simulink library "halin"  (R2021b)
settings: Solver=VariableStepAuto  StartTime=0.0  StopTime=10.0  RelTol=1e-3
undefined symbols (not defined in the file): KHAL_CAN1ABM1E2E_flg, KHAL_CAN1EPB1E2E_flg, KHAL_CAN1EPS1E2E_flg, KHAL_CAN1ESC1E2E_flg, KHAL_CAN1ESC5E2E_flg, KHAL_CAN3BMS1E2E_flg, KHAL_CAN3BMS6E2E_flg, KHAL_CAN3CCU1E2E_flg, KHAL_CAN3CCU2E2E_flg, KHAL_CAN3MCUNF1E2E_flg, KHAL_CAN3MCUNR1E2E_flg, KHAL_CAN3Shifter1E2E_flg, KHAL_CAN3Shifter2E2E_flg, KHAL_CAN6FCM2E2E_flg, KHAL_CAN6FCM4E2E_flg, TRUE
libraries: simulink x645, FVT_lib x207, hcu_lib x59
(part 6 of 23)

== system halin/HAL_IN/CAN1/EPS1 ==
  DT_CAN1_SG_EPS1 : Inport
  0x8E : Constant  Value=0x8E
  0xB1 : Constant  Value=0xB1
  BitwiseAND{,1..34} (35 alike) : simulink/Logic and Bit Operations/Bitwise Operator  logicop=AND  UseBitMask=on  BitMask=0xFF  BitMaskRealWorld=Stored Integer
  BitwiseOR{,1,4..6,8..10,12,14..15} (11 alike) : simulink/Logic and Bit Operations/Bitwise Operator  logicop=OR  UseBitMask=off  BitMask=bin2dec('11011001')  BitMaskRealWorld=Stored Integer
  BitwiseOR11 : simulink/Logic and Bit Operations/Bitwise Operator  logicop=OR  UseBitMask=off  NumInputPorts=6  BitMask=bin2dec('11011001')  BitMaskRealWorld=Stored Integer
  BitwiseOR13 : simulink/Logic and Bit Operations/Bitwise Operator  logicop=OR  UseBitMask=off  NumInputPorts=3  BitMask=bin2dec('11011001')  BitMaskRealWorld=Stored Integer
  BitwiseOR2 : simulink/Logic and Bit Operations/Bitwise Operator  logicop=OR  UseBitMask=off  NumInputPorts=6  BitMask=bin2dec('11011001')  BitMaskRealWorld=Stored Integer
  BitwiseOR3 : simulink/Logic and Bit Operations/Bitwise Operator  logicop=OR  UseBitMask=off  NumInputPorts=3  BitMask=bin2dec('11011001')  BitMaskRealWorld=Stored Integer
  BitwiseOR7 : simulink/Logic and Bit Operations/Bitwise Operator  logicop=OR  UseBitMask=off  NumInputPorts=6  BitMask=bin2dec('11011001')  BitMaskRealWorld=Stored Integer
  DDM_CS&RC_Comparison : FVT_lib/hal/DDM_CS&RC_Comparison  MsgCycleTime=10
  Data Type Conversion{,1..34} (35 alike) : DataTypeConversion  OutDataTypeStr=uint8
  DriIntend : Subsystem
  EPSAOIControl : Subsystem
  EPSRC : Subsystem
  EPSTOIActivation : Subsystem
  EPSTOIFault : Subsystem
  EPSTOIUnavailable : Subsystem
  EpasFailed : Subsystem
  KHAL_CAN1EPS1E2E_flg : Constant  Value=KHAL_CAN1EPS1E2E_flg
  LeftShift{,2,6..7} (4 alike) : ArithShift  BitShiftNumber=1  BitShiftDirection=Left
  LeftShift1 : ArithShift  BitShiftNumber=3  BitShiftDirection=Left
  LeftShift10 : ArithShift  BitShiftNumber=3  BitShiftDirection=Left
  LeftShift{3..4,11,15,17,21,23} (7 alike) : ArithShift  BitShiftDirection=Left
  LeftShift12 : ArithShift  BitShiftNumber=5  BitShiftDirection=Left
  LeftShift13 : ArithShift  BitShiftNumber=7  BitShiftDirection=Left
  LeftShift14 : ArithShift  BitShiftNumber=6  BitShiftDirection=Left
  LeftShift16 : ArithShift  BitShiftNumber=5  BitShiftDirection=Left
  LeftShift18 : ArithShift  BitShiftNumber=4  BitShiftDirection=Left
  LeftShift19 : ArithShift  BitShiftNumber=6  BitShiftDirection=Left
  LeftShift20 : ArithShift  BitShiftNumber=7  BitShiftDirection=Left
  LeftShift22 : ArithShift  BitShiftNumber=6  BitShiftDirection=Left
  LeftShift24 : ArithShift  BitShiftNumber=4  BitShiftDirection=Left
  LeftShift5 : ArithShift  BitShiftNumber=2  BitShiftDirection=Left
  LeftShift8 : ArithShift  BitShiftNumber=3  BitShiftDirection=Left
  LeftShift9 : ArithShift  BitShiftNumber=5  BitShiftDirection=Left
  MessageRollingCounter : FVT_lib/hal/MessageRollingCounter  CounterMAX=14  task_time_ms=5  msg_time_ms=10
  Mux : Mux  Inputs=15
  RightShift{,2,6,8} (4 alike) : ArithShift  BitShiftNumber=8
  RightShift{1,3,7,9} (4 alike) : ArithShift
  RightShift4 : ArithShift  BitShiftNumber=3
  RightShift5 : ArithShift  BitShiftNumber=-5
  SASAngle : Subsystem
  SASCAL : Subsystem
  SASSpeed : Subsystem
  SASSpeedValid : Subsystem
  SASV : Subsystem
  bus_selector : BusSelector  OutputSignals=CAN1_DriIntend,CAN1_EPS_AOI_Control,CAN1_EPS_AOI_Dis_R,CAN1_EPS_CS,CAN1_EPS_DMSMode_Sta,CAN1_EPS_ESABoostOut_Trq,CAN1_EPS_ESAInpBoost_Sta,CAN1_EPS_LDW_Activation,CAN1_EPS_LDW_Unavailable,CAN1_EPS_Pwr_Consumpt,CAN1_EPS_Pwr_Consumpt_V,CAN1_EPS_Pwr_Limit,CAN1_EPS_Pwr_Limit_V,CAN1_EPS_RC,CAN1_EPS_TOI_Activation,CAN1_EPS_TOI_Dis_R,CAN1_EPS_TOI_Fault,CAN1_EPS_TOI_Unavailable,CAN1_EPS_Temp,CAN1_EPS_Temp_V,CAN1_EPS_VOL,CAN1_EPS_VOL_V,CAN1_EpasFailed,CAN1_SAS_Angle,CAN1_SAS_CAL,CAN1_SAS_Speed,CAN1_SAS_Speed_Valid,CAN1_SAS_V,CAN1_Steering_Torque,CAN1_Steering_Torque_V
  bus_selector1 : BusSelector  OutputSignals=CAN1_DriIntend
  bus_selector10 : BusSelector  OutputSignals=CAN1_SAS_Speed
  bus_selector11 : BusSelector  OutputSignals=CAN1_SAS_Speed_Valid
  bus_selector12 : BusSelector  OutputSignals=CAN1_SAS_V
  bus_selector2 : BusSelector  OutputSignals=CAN1_EPS_AOI_Control
  bus_selector3 : BusSelector  OutputSignals=CAN1_EPS_RC
  bus_selector4 : BusSelector  OutputSignals=CAN1_EPS_TOI_Activation
  bus_selector5 : BusSelector  OutputSignals=CAN1_EPS_TOI_Fault
  bus_selector6 : BusSelector  OutputSignals=CAN1_EPS_TOI_Unavailable
  bus_selector7 : BusSelector  OutputSignals=CAN1_EpasFailed
  bus_selector8 : BusSelector  OutputSignals=CAN1_SAS_Angle
  bus_selector9 : BusSelector  OutputSignals=CAN1_SAS_CAL
  VHAL_EPS1CSErr_flg : Outport
  VHAL_EPS1RCErr_flg : Outport  Port=2
  VHAL_DriIntend_enum : Outport  Port=3
  VHAL_EPSAOIControl_enum : Outport  Port=4
  VHAL_EPSRC_enum : Outport  Port=5
  VHAL_EPSTOIActivation_flg : Outport  Port=6
  VHAL_EPSTOIFault_flg : Outport  Port=7
  VHAL_EPSTOIUnavailable_flg : Outport  Port=8
  VHAL_EpasFailed_enum : Outport  Port=9
  VHAL_SASAngle_Deg : Outport  Port=10
  VHAL_SASCAL_flg : Outport  Port=11
  VHAL_SASSpeed_degps : Outport  Port=12
  VHAL_SASSpeedValid_flg : Outport  Port=13
  VHAL_SASV_flg : Outport  Port=14
  wires:
  DT_CAN1_SG_EPS1/1 -> [DT_CAN1_SG_EPS1]
  [DT_CAN1_SG_EPS1] -> bus_selector/1
  bus_selector/1 -> [CAN1_DriIntend]  "<CAN1_DriIntend>"
  [CAN1_DriIntend] -> LeftShift/1
  LeftShift/1 -> BitwiseAND/1
  BitwiseAND/1 -> [Byte_2_CAN1_DriIntend]
  bus_selector/2 -> [CAN1_EPS_AOI_Control]  "<CAN1_EPS_AOI_Control>"
  [CAN1_EPS_AOI_Control] -> LeftShift1/1
  LeftShift1/1 -> BitwiseAND1/1
  BitwiseAND1/1 -> [Byte_2_CAN1_EPS_AOI_Control]
  bus_selector/3 -> [CAN1_EPS_AOI_Dis_R]  "<CAN1_EPS_AOI_Dis_R>"
  [CAN1_EPS_AOI_Dis_R] -> LeftShift2/1
  LeftShift2/1 -> BitwiseAND2/1
  BitwiseAND2/1 -> [Byte_3_CAN1_EPS_AOI_Dis_R]
  bus_selector/4 -> [CAN1_EPS_CS]  "<CAN1_EPS_CS>"
  [CAN1_EPS_CS] -> LeftShift3/1
  LeftShift3/1 -> BitwiseAND3/1
  BitwiseAND3/1 -> [Byte_0_CAN1_EPS_CS]
  bus_selector/5 -> [CAN1_EPS_DMSMode_Sta]  "<CAN1_EPS_DMSMode_Sta>"
  [CAN1_EPS_DMSMode_Sta] -> LeftShift4/1
  LeftShift4/1 -> BitwiseAND4/1
  BitwiseAND4/1 -> [Byte_15_CAN1_EPS_DMSMode_Sta]
  bus_selector/6 -> [CAN1_EPS_ESABoostOut_Trq]  "<CAN1_EPS_ESABoostOut_Trq>"
  [CAN1_EPS_ESABoostOut_Trq] -> LeftShift5/1
  LeftShift5/1 -> BitwiseAND5/1
  BitwiseAND5/1 -> [Byte_13_CAN1_EPS_ESABoostOut_Trq]
  bus_selector/7 -> [CAN1_EPS_ESAInpBoost_Sta]  "<CAN1_EPS_ESAInpBoost_Sta>"
  [CAN1_EPS_ESAInpBoost_Sta] -> LeftShift6/1
  LeftShift6/1 -> BitwiseAND6/1
  BitwiseAND6/1 -> [Byte_13_CAN1_EPS_ESAInpBoost_Sta]
  bus_selector/8 -> [CAN1_EPS_LDW_Activation]  "<CAN1_EPS_LDW_Activation>"
  [CAN1_EPS_LDW_Activation] -> LeftShift7/1
  LeftShift7/1 -> BitwiseAND7/1
  BitwiseAND7/1 -> [Byte_11_CAN1_EPS_LDW_Activation]
  bus_selector/9 -> [CAN1_EPS_LDW_Unavailable]  "<CAN1_EPS_LDW_Unavailable>"
  [CAN1_EPS_LDW_Unavailable] -> LeftShift8/1
  LeftShift8/1 -> BitwiseAND8/1
  BitwiseAND8/1 -> [Byte_11_CAN1_EPS_LDW_Unavailable]
  bus_selector/10 -> [CAN1_EPS_Pwr_Consumpt]  "<CAN1_EPS_Pwr_Consumpt>"
  [CAN1_EPS_Pwr_Consumpt] -> RightShift/1, RightShift1/1
  RightShift/1 -> BitwiseAND9/1
  BitwiseAND9/1 -> [Byte_13_CAN1_EPS_Pwr_Consumpt]
  RightShift1/1 -> BitwiseAND10/1
  BitwiseAND10/1 -> [Byte_14_CAN1_EPS_Pwr_Consumpt]
  bus_selector/11 -> [CAN1_EPS_Pwr_Consumpt_V]  "<CAN1_EPS_Pwr_Consumpt_V>"
  [CAN1_EPS_Pwr_Consumpt_V] -> LeftShift9/1
  LeftShift9/1 -> BitwiseAND11/1
  BitwiseAND11/1 -> [Byte_7_CAN1_EPS_Pwr_Consumpt_V]
  bus_selector/12 -> [CAN1_EPS_Pwr_Limit]  "<CAN1_EPS_Pwr_Limit>"
  [CAN1_EPS_Pwr_Limit] -> RightShift2/1, RightShift3/1
  RightShift2/1 -> BitwiseAND12/1
  BitwiseAND12/1 -> [Byte_11_CAN1_EPS_Pwr_Limit]
  RightShift3/1 -> BitwiseAND13/1
  BitwiseAND13/1 -> [Byte_12_CAN1_EPS_Pwr_Limit]
  bus_selector/13 -> [CAN1_EPS_Pwr_Limit_V]  "<CAN1_EPS_Pwr_Limit_V>"
  [CAN1_EPS_Pwr_Limit_V] -> LeftShift10/1
  LeftShift10/1 -> BitwiseAND14/1
  BitwiseAND14/1 -> [Byte_7_CAN1_EPS_Pwr_Limit_V]
  bus_selector/14 -> [CAN1_EPS_RC]  "<CAN1_EPS_RC>"
  [CAN1_EPS_RC] -> LeftShift11/1
  LeftShift11/1 -> BitwiseAND15/1
  BitwiseAND15/1 -> [Byte_1_CAN1_EPS_RC]
  bus_selector/15 -> [CAN1_EPS_TOI_Activation]  "<CAN1_EPS_TOI_Activation>"
  [CAN1_EPS_TOI_Activation] -> LeftShift12/1
  LeftShift12/1 -> BitwiseAND16/1
  BitwiseAND16/1 -> [Byte_2_CAN1_EPS_TOI_Activation]
  bus_selector/16 -> [CAN1_EPS_TOI_Dis_R]  "<CAN1_EPS_TOI_Dis_R>"
  [CAN1_EPS_TOI_Dis_R] -> RightShift4/1, RightShift5/1
  RightShift4/1 -> BitwiseAND17/1
  BitwiseAND17/1 -> [Byte_2_CAN1_EPS_TOI_Dis_R]
  RightShift5/1 -> BitwiseAND18/1
  BitwiseAND18/1 -> [Byte_3_CAN1_EPS_TOI_Dis_R]
  bus_selector/17 -> [CAN1_EPS_TOI_Fault]  "<CAN1_EPS_TOI_Fault>"
  [CAN1_EPS_TOI_Fault] -> LeftShift13/1
  LeftShift13/1 -> BitwiseAND19/1
  BitwiseAND19/1 -> [Byte_2_CAN1_EPS_TOI_Fault]
  bus_selector/18 -> [CAN1_EPS_TOI_Unavailable]  "<CAN1_EPS_TOI_Unavailable>"
  [CAN1_EPS_TOI_Unavailable] -> LeftShift14/1
  LeftShift14/1 -> BitwiseAND20/1
  BitwiseAND20/1 -> [Byte_2_CAN1_EPS_TOI_Unavailable]
  bus_selector/19 -> [CAN1_EPS_Temp]  "<CAN1_EPS_Temp>"
  [CAN1_EPS_Temp] -> LeftShift15/1
  LeftShift15/1 -> BitwiseAND21/1
  BitwiseAND21/1 -> [Byte_10_CAN1_EPS_Temp]
  bus_selector/20 -> [CAN1_EPS_Temp_V]  "<CAN1_EPS_Temp_V>"
  [CAN1_EPS_Temp_V] -> LeftShift16/1
  LeftShift16/1 -> BitwiseAND22/1
  BitwiseAND22/1 -> [Byte_11_CAN1_EPS_Temp_V]
  bus_selector/21 -> [CAN1_EPS_VOL]  "<CAN1_EPS_VOL>"
  [CAN1_EPS_VOL] -> LeftShift17/1
  LeftShift17/1 -> BitwiseAND23/1
  BitwiseAND23/1 -> [Byte_9_CAN1_EPS_VOL]
  bus_selector/22 -> [CAN1_EPS_VOL_V]  "<CAN1_EPS_VOL_V>"
  [CAN1_EPS_VOL_V] -> LeftShift18/1
  LeftShift18/1 -> BitwiseAND24/1
  BitwiseAND24/1 -> [Byte_11_CAN1_EPS_VOL_V]
  bus_selector/23 -> [CAN1_EpasFailed]  "<CAN1_EpasFailed>"
  [CAN1_EpasFailed] -> LeftShift19/1
  LeftShift19/1 -> BitwiseAND25/1
  BitwiseAND25/1 -> [Byte_11_CAN1_EpasFailed]
  bus_selector/24 -> [CAN1_SAS_Angle]  "<CAN1_SAS_Angle>"
  [CAN1_SAS_Angle] -> RightShift6/1, RightShift7/1
  RightShift6/1 -> BitwiseAND26/1
  BitwiseAND26/1 -> [Byte_5_CAN1_SAS_Angle]
  RightShift7/1 -> BitwiseAND27/1
  BitwiseAND27/1 -> [Byte_6_CAN1_SAS_Angle]
  bus_selector/25 -> [CAN1_SAS_CAL]  "<CAN1_SAS_CAL>"
  [CAN1_SAS_CAL] -> LeftShift20/1
  LeftShift20/1 -> BitwiseAND28/1
  BitwiseAND28/1 -> [Byte_7_CAN1_SAS_CAL]
  bus_selector/26 -> [CAN1_SAS_Speed]  "<CAN1_SAS_Speed>"
  [CAN1_SAS_Speed] -> LeftShift21/1
  LeftShift21/1 -> BitwiseAND29/1
  BitwiseAND29/1 -> [Byte_4_CAN1_SAS_Speed]
  bus_selector/27 -> [CAN1_SAS_Speed_Valid]  "<CAN1_SAS_Speed_Valid>"
  [CAN1_SAS_Speed_Valid] -> LeftShift22/1
  LeftShift22/1 -> BitwiseAND30/1
  BitwiseAND30/1 -> [Byte_7_CAN1_SAS_Speed_Valid]
  bus_selector/28 -> [CAN1_SAS_V]  "<CAN1_SAS_V>"
  [CAN1_SAS_V] -> LeftShift23/1
  LeftShift23/1 -> BitwiseAND31/1
  BitwiseAND31/1 -> [Byte_3_CAN1_SAS_V]
  bus_selector/29 -> [CAN1_Steering_Torque]  "<CAN1_Steering_Torque>"
  [CAN1_Steering_Torque] -> RightShift8/1, RightShift9/1
  RightShift8/1 -> BitwiseAND32/1
  BitwiseAND32/1 -> [Byte_7_CAN1_Steering_Torque]
  RightShift9/1 -> BitwiseAND33/1
  BitwiseAND33/1 -> [Byte_8_CAN1_Steering_Torque]
  bus_selector/30 -> [CAN1_Steering_Torque_V]  "<CAN1_Steering_Torque_V>"
  [CAN1_Steering_Torque_V] -> LeftShift24/1
  LeftShift24/1 -> BitwiseAND34/1
  BitwiseAND34/1 -> [Byte_7_CAN1_Steering_Torque_V]
  Data Type Conversion/1 -> BitwiseOR/1
  [Byte_0_CAN1_EPS_CS] -> Data Type Conversion/1
  BitwiseOR/1 -> [Byte_0]
  Data Type Conversion1/1 -> BitwiseOR1/1
  [Byte_1_CAN1_EPS_RC] -> Data Type Conversion1/1
  BitwiseOR1/1 -> [Byte_1]
  Data Type Conversion2/1 -> BitwiseOR2/1
  [Byte_2_CAN1_DriIntend] -> Data Type Conversion2/1
  Data Type Conversion3/1 -> BitwiseOR2/2
  [Byte_2_CAN1_EPS_AOI_Control] -> Data Type Conversion3/1
  Data Type Conversion4/1 -> BitwiseOR2/3
  [Byte_2_CAN1_EPS_TOI_Activation] -> Data Type Conversion4/1
  Data Type Conversion5/1 -> BitwiseOR2/4
  [Byte_2_CAN1_EPS_TOI_Dis_R] -> Data Type Conversion5/1
  Data Type Conversion6/1 -> BitwiseOR2/5
  [Byte_2_CAN1_EPS_TOI_Fault] -> Data Type Conversion6/1
  Data Type Conversion7/1 -> BitwiseOR2/6
  [Byte_2_CAN1_EPS_TOI_Unavailable] -> Data Type Conversion7/1
  BitwiseOR2/1 -> [Byte_2]
  Data Type Conversion8/1 -> BitwiseOR3/1
  [Byte_3_CAN1_EPS_AOI_Dis_R] -> Data Type Conversion8/1
  Data Type Conversion9/1 -> BitwiseOR3/2
  [Byte_3_CAN1_EPS_TOI_Dis_R] -> Data Type Conversion9/1
  Data Type Conversion10/1 -> BitwiseOR3/3
  [Byte_3_CAN1_SAS_V] -> Data Type Conversion10/1
  BitwiseOR3/1 -> [Byte_3]
  Data Type Conversion11/1 -> BitwiseOR4/1
  [Byte_4_CAN1_SAS_Speed] -> Data Type Conversion11/1
  BitwiseOR4/1 -> [Byte_4]
  Data Type Conversion12/1 -> BitwiseOR5/1
  [Byte_5_CAN1_SAS_Angle] -> Data Type Conversion12/1
  BitwiseOR5/1 -> [Byte_5]
  Data Type Conversion13/1 -> BitwiseOR6/1
  [Byte_6_CAN1_SAS_Angle] -> Data Type Conversion13/1
  BitwiseOR6/1 -> [Byte_6]
  Data Type Conversion14/1 -> BitwiseOR7/1
  [Byte_7_CAN1_EPS_Pwr_Consumpt_V] -> Data Type Conversion14/1
  Data Type Conversion15/1 -> BitwiseOR7/2
  [Byte_7_CAN1_EPS_Pwr_Limit_V] -> Data Type Conversion15/1
  Data Type Conversion16/1 -> BitwiseOR7/3
  [Byte_7_CAN1_SAS_CAL] -> Data Type Conversion16/1
  Data Type Conversion17/1 -> BitwiseOR7/4
  [Byte_7_CAN1_SAS_Speed_Valid] -> Data Type Conversion17/1
  Data Type Conversion18/1 -> BitwiseOR7/5
  [Byte_7_CAN1_Steering_Torque] -> Data Type Conversion18/1
  Data Type Conversion19/1 -> BitwiseOR7/6
  [Byte_7_CAN1_Steering_Torque_V] -> Data Type Conversion19/1
  BitwiseOR7/1 -> [Byte_7]
  Data Type Conversion20/1 -> BitwiseOR8/1
  [Byte_8_CAN1_Steering_Torque] -> Data Type Conversion20/1
  BitwiseOR8/1 -> [Byte_8]
  Data Type Conversion21/1 -> BitwiseOR9/1
  [Byte_9_CAN1_EPS_VOL] -> Data Type Conversion21/1
  BitwiseOR9/1 -> [Byte_9]
  Data Type Conversion22/1 -> BitwiseOR10/1
  [Byte_10_CAN1_EPS_Temp] -> Data Type Conversion22/1
  BitwiseOR10/1 -> [Byte_10]
  Data Type Conversion23/1 -> BitwiseOR11/1
  [Byte_11_CAN1_EPS_LDW_Activation] -> Data Type Conversion23/1
  Data Type Conversion24/1 -> BitwiseOR11/2
  [Byte_11_CAN1_EPS_LDW_Unavailable] -> Data Type Conversion24/1
  Data Type Conversion25/1 -> BitwiseOR11/3
  [Byte_11_CAN1_EPS_Pwr_Limit] -> Data Type Conversion25/1
  Data Type Conversion26/1 -> BitwiseOR11/4
  [Byte_11_CAN1_EPS_Temp_V] -> Data Type Conversion26/1
  Data Type Conversion27/1 -> BitwiseOR11/5
  [Byte_11_CAN1_EPS_VOL_V] -> Data Type Conversion27/1
  Data Type Conversion28/1 -> BitwiseOR11/6
  [Byte_11_CAN1_EpasFailed] -> Data Type Conversion28/1
  BitwiseOR11/1 -> [Byte_11]
  Data Type Conversion29/1 -> BitwiseOR12/1
  [Byte_12_CAN1_EPS_Pwr_Limit] -> Data Type Conversion29/1
  BitwiseOR12/1 -> [Byte_12]
  Data Type Conversion30/1 -> BitwiseOR13/1
  [Byte_13_CAN1_EPS_ESABoostOut_Trq] -> Data Type Conversion30/1
  Data Type Conversion31/1 -> BitwiseOR13/2
  [Byte_13_CAN1_EPS_ESAInpBoost_Sta] -> Data Type Conversion31/1
  Data Type Conversion32/1 -> BitwiseOR13/3
  [Byte_13_CAN1_EPS_Pwr_Consumpt] -> Data Type Conversion32/1
  BitwiseOR13/1 -> [Byte_13]
  Data Type Conversion33/1 -> BitwiseOR14/1
  [Byte_14_CAN1_EPS_Pwr_Consumpt] -> Data Type Conversion33/1
  BitwiseOR14/1 -> [Byte_14]
  Data Type Conversion34/1 -> BitwiseOR15/1
  [Byte_15_CAN1_EPS_DMSMode_Sta] -> Data Type Conversion34/1
  BitwiseOR15/1 -> [Byte_15]
  [Byte_1] -> Mux/1
  [Byte_2] -> Mux/2
  [Byte_3] -> Mux/3
  [Byte_4] -> Mux/4
  [Byte_5] -> Mux/5
  [Byte_6] -> Mux/6
  [Byte_7] -> Mux/7
  [Byte_8] -> Mux/8
  [Byte_9] -> Mux/9
  [Byte_10] -> Mux/10
  [Byte_11] -> Mux/11
  [Byte_12] -> Mux/12
  [Byte_13] -> Mux/13
  [Byte_14] -> Mux/14
  [Byte_15] -> Mux/15
  Mux/1 -> [VHAL_CAN1EPS1noCS_raw]
  KHAL_CAN1EPS1E2E_flg/1 -> DDM_CS&RC_Comparison/1
  0x8E/1 -> DDM_CS&RC_Comparison/2
  0xB1/1 -> DDM_CS&RC_Comparison/3
  [VHAL_CAN1EPS1noCS_raw] -> DDM_CS&RC_Comparison/4
  [Byte_0] -> DDM_CS&RC_Comparison/5
  [RC_ECU] -> DDM_CS&RC_Comparison/6
  MessageRollingCounter/1 -> DDM_CS&RC_Comparison/7
  DDM_CS&RC_Comparison/1 -> VHAL_EPS1CSErr_flg/1
  DDM_CS&RC_Comparison/2 -> VHAL_EPS1RCErr_flg/1
  [DT_CAN1_SG_EPS1] -> bus_selector1/1
  bus_selector1/1 -> DriIntend/1(DriIntend)  "<CAN1_DriIntend>"
  DriIntend/1(VHAL_DriIntend_enum) -> VHAL_DriIntend_enum/1
  [DT_CAN1_SG_EPS1] -> bus_selector2/1
  bus_selector2/1 -> EPSAOIControl/1(EPS_AOI_Control)  "<CAN1_EPS_AOI_Control>"
  EPSAOIControl/1(VHAL_EPSAOIControl_enum) -> VHAL_EPSAOIControl_enum/1
  [DT_CAN1_SG_EPS1] -> bus_selector3/1
  bus_selector3/1 -> EPSRC/1(EPS_RC)  "<CAN1_EPS_RC>"
  EPSRC/1(VHAL_EPSRC_enum) -> VHAL_EPSRC_enum/1, [RC_ECU]
  [DT_CAN1_SG_EPS1] -> bus_selector4/1
  bus_selector4/1 -> EPSTOIActivation/1(EPS_TOI_Activation)  "<CAN1_EPS_TOI_Activation>"
  EPSTOIActivation/1(VHAL_EPSTOIActivation_flg) -> VHAL_EPSTOIActivation_flg/1
  [DT_CAN1_SG_EPS1] -> bus_selector5/1
  bus_selector5/1 -> EPSTOIFault/1(EPS_TOI_Fault)  "<CAN1_EPS_TOI_Fault>"
  EPSTOIFault/1(VHAL_EPSTOIFault_flg) -> VHAL_EPSTOIFault_flg/1
  [DT_CAN1_SG_EPS1] -> bus_selector6/1
  bus_selector6/1 -> EPSTOIUnavailable/1(EPS_TOI_Unavailable)  "<CAN1_EPS_TOI_Unavailable>"
  EPSTOIUnavailable/1(VHAL_EPSTOIUnavailable_flg) -> VHAL_EPSTOIUnavailable_flg/1
  [DT_CAN1_SG_EPS1] -> bus_selector7/1
  bus_selector7/1 -> EpasFailed/1(EpasFailed)  "<CAN1_EpasFailed>"
  EpasFailed/1(VHAL_EpasFailed_enum) -> VHAL_EpasFailed_enum/1
  [DT_CAN1_SG_EPS1] -> bus_selector8/1
  bus_selector8/1 -> SASAngle/1(SAS_Angle)  "<CAN1_SAS_Angle>"
  SASAngle/1(VHAL_SASAngle_Deg) -> VHAL_SASAngle_Deg/1
  [DT_CAN1_SG_EPS1] -> bus_selector9/1
  bus_selector9/1 -> SASCAL/1(SAS_CAL)  "<CAN1_SAS_CAL>"
  SASCAL/1(VHAL_SASCAL_flg) -> VHAL_SASCAL_flg/1
  [DT_CAN1_SG_EPS1] -> bus_selector10/1
  bus_selector10/1 -> SASSpeed/1(SAS_Speed)  "<CAN1_SAS_Speed>"
  SASSpeed/1(VHAL_SASSpeed_degps) -> VHAL_SASSpeed_degps/1
  [DT_CAN1_SG_EPS1] -> bus_selector11/1
  bus_selector11/1 -> SASSpeedValid/1(SAS_Speed_Valid)  "<CAN1_SAS_Speed_Valid>"
  SASSpeedValid/1(VHAL_SASSpeedValid_flg) -> VHAL_SASSpeedValid_flg/1
  [DT_CAN1_SG_EPS1] -> bus_selector12/1
  bus_selector12/1 -> SASV/1(SAS_V)  "<CAN1_SAS_V>"
  SASV/1(VHAL_SASV_flg) -> VHAL_SASV_flg/1
